simulink model "systemModel_Final"  (R2015a)
settings: Solver=ode3  StartTime=0.0  StopTime=3  FixedStep=0.01  RelTol=1e-3
libraries: fuzblock x1
settings Model: Creator=Φίλιππος  LastModifiedBy=ALKATRAZ
settings ConfigComp: Description=Design Verifier Custom Configuration Component  DVMaxTestCaseSteps=500  DVTestSuiteOptimization=CombinedObjectives (Nonlinear Extended)

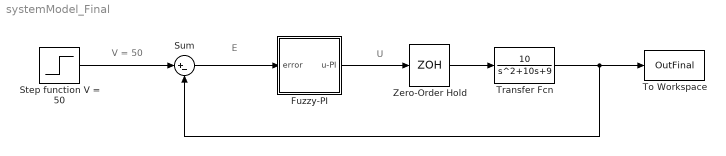
== system systemModel_Final ==
  note: U
  note: E
  note: V = 50
  Fuzzy-PI : Subsystem
  Step function V = 50 : Step  Time=0  After=50  SampleTime=0  ZeroCross=off
  Sum : Sum  Inputs=|+-
  To Workspace : ToWorkspace  VariableName=OutFinal  SaveFormat=Timeseries  SampleTime=-1
  Transfer Fcn : TransferFcn  Numerator=[10]  Denominator=[1 10 9]
  Zero-Order Hold : ZeroOrderHold  SampleTime=0.01
  wires:
  Zero-Order Hold/1 -> Transfer Fcn/1
  Step function V = 50/1 -> Sum/1
  Transfer Fcn/1 -> To Workspace/1, Sum/2
  Fuzzy-PI/1(u-PI) -> Zero-Order Hold/1
  Sum/1 -> Fuzzy-PI/1(error)

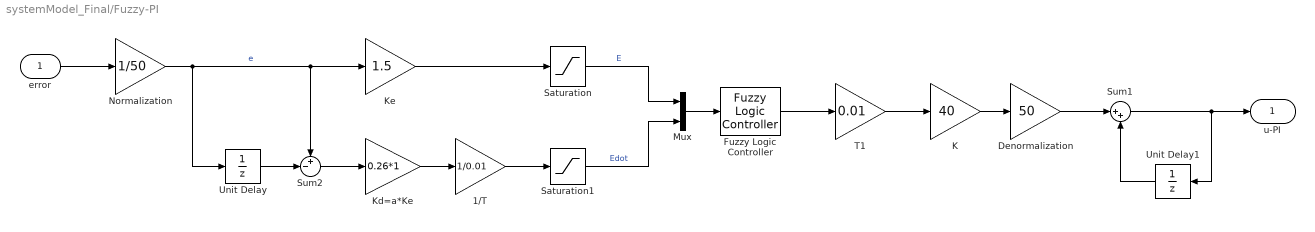
== system systemModel_Final/Fuzzy-PI ==
  error : Inport
  1/T : Gain  Gain=1/0.01
  Denormalization : Gain  Gain=50
  Fuzzy Logic Controller : fuzblock/Fuzzy Logic  Controller  fis='FuzzyController.fis'
  K : Gain  Gain=40
  Kd=a*Ke : Gain  Gain=0.26*1
  Ke : Gain  Gain=1.5
  Mux : Mux  Inputs=2
  Normalization : Gain  Gain=1/50
  Saturation : Saturate  UpperLimit=1  LowerLimit=-1
  Saturation1 : Saturate  UpperLimit=1  LowerLimit=-1
  Sum1 : Sum  Inputs=|++
  Sum2 : Sum  Inputs=+-|
  T1 : Gain  Gain=0.01
  Unit Delay : UnitDelay  SampleTime=-1
  Unit Delay1 : UnitDelay  SampleTime=-1
  u-PI : Outport
  wires:
  error/1 -> Normalization/1
  Normalization/1 -> Unit Delay/1, Sum2/1, Ke/1  "e"
  Unit Delay/1 -> Sum2/2
  Ke/1 -> Saturation/1
  Kd=a*Ke/1 -> 1/T/1
  1/T/1 -> Saturation1/1
  Saturation/1 -> Mux/1  "E"
  Saturation1/1 -> Mux/2  "Edot"
  Mux/1 -> Fuzzy Logic Controller/1
  Fuzzy Logic Controller/1 -> T1/1
  T1/1 -> K/1
  K/1 -> Denormalization/1
  Denormalization/1 -> Sum1/1
  Sum1/1 -> Unit Delay1/1, u-PI/1
  Unit Delay1/1 -> Sum1/2
  Sum2/1 -> Kd=a*Ke/1
